simulink model "DC_Motor_Simscape_ClosedLoop"  (R2026a)
settings: Solver=ode23t  StopTime=0.5  MaxStep=5e-5
libraries: fl_lib x6, nesl_utility x4, ee_lib x1
settings Model: Creator=PattarapolSangaroon  LastModifiedBy=PattarapolSangaroon
settings DataIOCC: OutputSaveName=motorOutputs

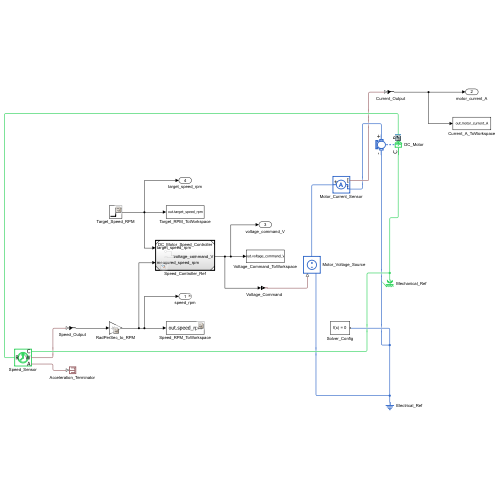
[thumbnail: Simulink's stored preview of the top-level diagram]
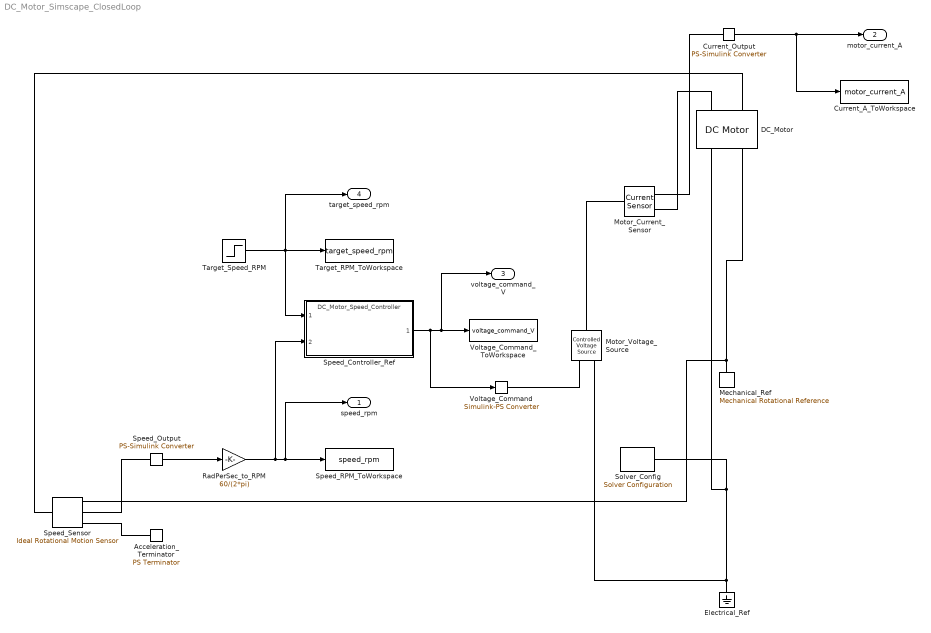
== system DC_Motor_Simscape_ClosedLoop ==
  Acceleration_Terminator : fl_lib/Physical Signals/Sinks/PS Terminator
  Current_A_ToWorkspace : ToWorkspace  VariableName=motor_current_A  SaveFormat=Timeseries  SampleTime=-1
  Current_Output : nesl_utility/PS-Simulink Converter  PhysicalDomain=network_engine_domain  SubClassName=ps_output  LeftPortType=input  RightPortType=output  PseudoPeriodic=off  Frequencies=[]  VectorFormat=inherit  Unit=A  AffineConversion=off
  DC_Motor : ee_lib/Electromechanical/Brushed Motors/DC Motor  field_option=ee.enum.field_option.pm  Rf=100 Ohm  Lf=1 H  Laf=0.15 H  If0=0 A  parameterization=ee.enum.dcparam_option.circuit_param  Ra=3.9 Ohm  La=12e-6 H  emf_or_torque=ee.enum.emf_or_torque.kv  Kv=0.012 V/rpm  Ki=6.876e-4 N*m/A  T_stall=0.24e-3 N*m  w_max=1200 rpm  w_rated=1000 rpm  P_rated=0.08 W  V_rated=12 V  lam_param=ee.enum.lam_param.damping  i_noload=0 A  V_i_noload=12 V  J=100 cm^2*g  lam=1e-5 N*m*s/rad  speed0=0 rpm  alpha=3.93e-3 1/K  Tmeas=25 degC  thermal_mass=100 J/K  initial_temperature=25 degC
  Electrical_Ref : fl_lib/Electrical/Electrical Elements/Electrical Reference
  Mechanical_Ref : fl_lib/Mechanical/Rotational Elements/Mechanical Rotational Reference
  Motor_Current_Sensor : fl_lib/Electrical/Electrical Sensors/Current Sensor
  Motor_Voltage_Source : fl_lib/Electrical/Electrical Sources/Controlled Voltage Source
  RadPerSec_to_RPM : Gain  Gain=60/(2*pi)
  Solver_Config : nesl_utility/Solver Configuration  PhysicalDomain=network_engine_domain  SubClassName=solver  LeftPortType=input  RightPortType=generic  Tones=[]  Harmonics=[]  SimulateNoise=off  Profile=off  UseLocalSampling=off  EnableSwitchedLinearOptims=on  FrequencyDomain=off  UseCCode=off  RelTol=0.001  AbsTol=0.001  MinStep=1e-09  ToWorkspace=off  RevertToSquareIcSolve=off  NumHomotopyIterations=100  PhasorMode=off  PhasorModeNumHarmonics=1  ConsistencySolver=NEWTON_XTOL_AFTER_FTOL  CanonicalOrdering=CANONICAL  OptimizeIntermediates=OPTIMIZED  IndexReductionMethod=DerivativeReplacement  DoDC=off  ResidualTolerance=1e-09  ConsistencyTolSource=GLOBAL  ConsistencyAbsTol=0.001  ConsistencyRelTol=0.001  ConsistencyTolFactor=0.001  UseLocalSolver=off  LocalSolverChoice=NE_BACKWARD_EULER_ADVANCER  ResolveIndetEquations=on  FunctionEvalNumThread=1  LocalSolverSampleTime=0.001  DoFixedCost=off  MaxNonlinIter=3  MaxModeIter=2  ComputeImpulses=off  ImpulseIterations=2  LinearAlgebra=auto  LinearAlgebraNumThread=0  EquationFormulation=NE_TIME_EF  DelaysMemoryBudget=1024  AutomaticFiltering=on  FilteringTimeConstant=0.001  PartitionStorageMethod=AS_NEEDED  PartitionMemoryBudget=1024  PartitionMethod=ROBUST  MultibodyUseLocalSolver=off  MultibodyLocalSolverChoice=ODE1  MultibodyLocalSolverSampleTime=0.001
  Speed_Controller_Ref : ModelReference  ModelNameDialog=DC_Motor_Speed_Controller  SimulationMode=Normal  ModelReferenceVersion=1.2
  Speed_Output : nesl_utility/PS-Simulink Converter  PhysicalDomain=network_engine_domain  SubClassName=ps_output  LeftPortType=input  RightPortType=output  PseudoPeriodic=off  Frequencies=[]  VectorFormat=inherit  Unit=rad/s  AffineConversion=off
  Speed_RPM_ToWorkspace : ToWorkspace  VariableName=speed_rpm  SaveFormat=Timeseries  SampleTime=-1
  Speed_Sensor : fl_lib/Mechanical/Mechanical Sensors/Ideal Rotational Motion Sensor  reference=foundation.enum.MeasurementReference.difference  acceleration_port=false  velocity_port=true  position_port=true  wrap_angle=false  offset=0 rad
  Target_RPM_ToWorkspace : ToWorkspace  VariableName=target_speed_rpm  SaveFormat=Timeseries  SampleTime=-1
  Target_Speed_RPM : Step  Time=0.05  FinalValue=600  SampleTime=0
  Voltage_Command : nesl_utility/Simulink-PS Converter  PhysicalDomain=network_engine_domain  SubClassName=ps_input  LeftPortType=input  RightPortType=output  PseudoPeriodic=off  Frequencies=[]  NoiseDistribution=none  NoiseParameters=[]  Unit=V  AffineConversion=off  FilteringAndDerivatives=provide  SimscapeFilterOrder=1  InputFilterTimeConstant=0.001  UdotUserProvided=0
  Voltage_Command_ToWorkspace : ToWorkspace  VariableName=voltage_command_V  SaveFormat=Timeseries  SampleTime=-1
  speed_rpm : Outport
  motor_current_A : Outport  Port=2
  voltage_command_V : Outport  Port=3
  target_speed_rpm : Outport  Port=4
  wires:
  Speed_Controller_Ref/1 -> Voltage_Command_ToWorkspace/1, voltage_command_V/1, Voltage_Command/1
  Target_Speed_RPM/1 -> target_speed_rpm/1, Target_RPM_ToWorkspace/1, Speed_Controller_Ref/1
  Current_Output/1 -> motor_current_A/1, Current_A_ToWorkspace/1
  Speed_Output/1 -> RadPerSec_to_RPM/1
  RadPerSec_to_RPM/1 -> speed_rpm/1, Speed_RPM_ToWorkspace/1, Speed_Controller_Ref/2
  connections:
  Motor_Voltage_Source/LConn1 -- Motor_Current_Sensor/LConn1
  Motor_Current_Sensor/RConn2 -- DC_Motor/LConn1
  Solver_Config/RConn1 -- Motor_Voltage_Source/RConn2 -- Electrical_Ref/LConn1 -- DC_Motor/RConn1
  DC_Motor/LConn2 -- Speed_Sensor/LConn1
  Speed_Sensor/RConn1 -- Mechanical_Ref/LConn1 -- DC_Motor/RConn2
  Voltage_Command/RConn1 -- Motor_Voltage_Source/RConn1
  Motor_Current_Sensor/RConn1 -- Current_Output/LConn1
  Speed_Sensor/RConn2 -- Speed_Output/LConn1
  Speed_Sensor/RConn3 -- Acceleration_Terminator/LConn1
